simulink model "exple_12102017"  (R2016b)
settings: Solver=VariableStepAuto  StartTime=0.0  StopTime=2  RelTol=1e-3
settings Model: Creator=live  LastModifiedBy=live

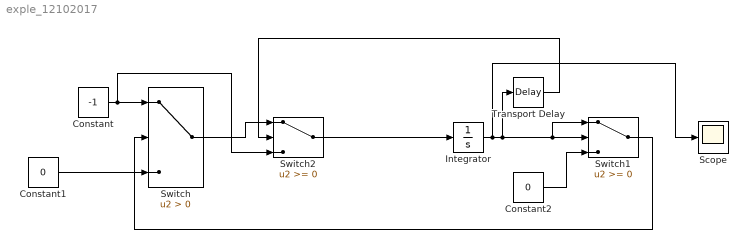
== system exple_12102017 ==
  Constant : Constant  Value=-1
  Constant1 : Constant  Value=0
  Constant2 : Constant  Value=0
  Integrator : Integrator  InitialCondition=1
  Scope : Scope
  Switch : Switch  Criteria=u2 > Threshold
  Switch1 : Switch
  Switch2 : Switch
  Transport Delay : TransportDelay  DelayTime=0.2  InitialOutput=1
  wires:
  Constant1/1 -> Switch/3
  Integrator/1 -> Scope/1, Transport Delay/1, Switch1/1, Switch1/2
  Constant2/1 -> Switch1/3
  Constant/1 -> Switch2/3, Switch/1
  Switch1/1 -> Switch/2
  Transport Delay/1 -> Switch2/2
  Switch/1 -> Switch2/1
  Switch2/1 -> Integrator/1
